simulink model "NoC_4x4x3"  (R2015a)
settings: Solver=ode45  StartTime=0.0  StopTime=10.0  RelTol=1e-3
undefined symbols (not defined in the file or in its folder): des, SELECT
undefined symbols (not defined in the file): MAX, MIN, T
libraries: simulink x48
(part 6 of 12)

== system NoC_4x4x3/LayerDown/PE10 ==
  Cancel Timeout : CancelTimeout
  Constant : Constant  Value=SELECT
  Create Generator Selection Variable : Subsystem  TreatAsAtomicUnit=on
      settings: PropExecContextOutsideSubsystem=on
  DST : EventBasedRandomNumber  Distribution=Arbitrary discrete  minUnid=1  maxUnid=16  numValueUnid=5  valueVecDisc=[1 2 3 4]  probVecDisc=[.25 .25 .25 .25]  Seed=SEED+5
  DST1 : EventBasedRandomNumber  Distribution=Arbitrary discrete  minUnid=1  maxUnid=16  numValueUnid=5  valueVecDisc=[1 2 3 4]  probVecDisc=[.25 .25 .25 .25]  Seed=SEED+50
  DST2 : EventBasedRandomNumber  Distribution=Arbitrary discrete  minUnid=1  maxUnid=16  numValueUnid=5  valueVecDisc=[1 2 3 4]  probVecDisc=[.25 .25 .25 .25]  Seed=SEED+500
  Enabled Gate : EnabledGate
  Entity Departure Event to Function-Call Event : EntityDepartureFunctionCallGenerator
  Entity Sink : EntitySink
  Entity Sink1 : EntitySink
  Entity Sink2 : EntitySink
  Generator 1 : TimeBasedEntityGenerator  Distribution=Exponential  Period=.1  InitialSeed=SEED+10  Maximum=.2  Mean=B  ResponseWhenUnblocked=Delayed restart  EntityType=Standard
  Infinite Server : InfiniteServer  ServiceTime=D  EnableTOPort=on
  Input Switch : InputSwitch  SwitchingCriterion=From signal port p
  Schedule Timeout : ScheduleTimeout  TimeoutInterval=D
  Set Attribute : SetAttribute  AttributeName=DST_X|DST_Y|DST_Z  AttributeFrom=Signal port|Signal port|Signal port  AttributeValue=16|1|1  AttributeTreatAsVector=0|1|1  EvaluatedAttributeValue={ [];[];[]}
      settings: InputPortMap=u0,u1,u2
  Start Timer : StartTimer  TimerTag=Departure
  Time-Based Entity Generator : TimeBasedEntityGenerator  Distribution=Exponential  Period=15  InitialSeed=51335  Maximum=2  Mean=A  PriorityEntityGeneration=350  EntityType=Standard
  Time-Based Entity Generator1 : TimeBasedEntityGenerator  Period=REGULAR
  Time-Based Entity Generator2 : TimeBasedEntityGenerator  Distribution=Uniform  InitialSeed=54552  Minimum=MINU  Maximum=MAXU
  Data_out : PMIOPort  Port=1  Side=Right
  Data_in : PMIOPort  Port=2  Side=Left
  wires:
  Create Generator Selection Variable/1(Out1) -> Enabled Gate/1
  Entity Departure Event to Function-Call Event/1 -> Create Generator Selection Variable/Trigger
  Constant/1 -> Input Switch/1
  DST/1 -> Set Attribute/1
  DST1/1 -> Set Attribute/2
  DST2/1 -> Set Attribute/3
  connections:
  Entity Departure Event to Function-Call Event/RConn1 -- Entity Sink/LConn1
  Time-Based Entity Generator/RConn1 -- Entity Departure Event to Function-Call Event/LConn1
  Generator 1/RConn1 -- Enabled Gate/LConn1
  Time-Based Entity Generator1/RConn1 -- Input Switch/LConn1
  Input Switch/LConn2 -- Time-Based Entity Generator2/RConn1
  Enabled Gate/RConn1 -- Input Switch/LConn3
  Schedule Timeout/LConn1 -- Set Attribute/RConn1
  Cancel Timeout/LConn1 -- Infinite Server/RConn1
  Set Attribute/LConn1 -- Input Switch/RConn1
  Data_out/RConn1 -- Start Timer/RConn1
  Start Timer/LConn1 -- Cancel Timeout/RConn1
  Entity Sink1/LConn1 -- Data_in/RConn1
  Schedule Timeout/RConn1 -- Infinite Server/LConn1
  Infinite Server/RConn2 -- Entity Sink2/LConn1

== system NoC_4x4x3/LayerDown/PE11 ==
  Constant : Constant  Value=SELECT
  Create Generator Selection Variable : Subsystem  TreatAsAtomicUnit=on
      settings: PropExecContextOutsideSubsystem=on
  DST : EventBasedRandomNumber  Distribution=Arbitrary discrete  minUnid=1  maxUnid=16  numValueUnid=5  valueVecDisc=[1 2 3 4]  probVecDisc=[.25 .25 .25 .25]  Seed=SEED+5
  DST1 : EventBasedRandomNumber  Distribution=Arbitrary discrete  minUnid=1  maxUnid=16  numValueUnid=5  valueVecDisc=[1 2 3 4]  probVecDisc=[.25 .25 .25 .25]  Seed=SEED+50
  DST2 : EventBasedRandomNumber  Distribution=Arbitrary discrete  minUnid=1  maxUnid=16  numValueUnid=5  valueVecDisc=[1 2 3 4]  probVecDisc=[.25 .25 .25 .25]  Seed=SEED+500
  Enabled Gate : EnabledGate
  Entity Departure Event to Function-Call Event : EntityDepartureFunctionCallGenerator
  Entity Sink : EntitySink
  Entity Sink1 : EntitySink
  Generator 1 : TimeBasedEntityGenerator  Distribution=Exponential  Period=.1  InitialSeed=SEED+10  Maximum=.2  Mean=B  ResponseWhenUnblocked=Delayed restart  EntityType=Standard
  Infinite Server : InfiniteServer  ServiceTime=0  StatAverageWait=on
      settings: OutputPortMap=o4
  Input Switch : InputSwitch  SwitchingCriterion=From signal port p  StatNumberDeparted=on
  Loss : ToWorkspace  VariableName=Midlle_Loss_Z1  SaveFormat=Timeseries  SampleTime=-1
  N : ToWorkspace  VariableName=Midlle_N_Z1  SaveFormat=Timeseries  SampleTime=-1
  Read Timer : ReadTimer  TimerTag=Departure  StatAverageTimeElapsed=on
      settings: OutputPortMap=o3
  Router : ToWorkspace  VariableName=Midlle_Mean_Z1  SaveFormat=Timeseries  SampleTime=-1
  Set Attribute : SetAttribute  AttributeName=DST_X|DST_Y|DST_Z  AttributeFrom=Signal port|Signal port|Signal port  AttributeValue=16|1|1  AttributeTreatAsVector=0|1|1  StatNumberDeparted=on  EvaluatedAttributeValue={ [];[];[]}
      settings: InputPortMap=u0,u1,u2
  Start Timer : StartTimer  TimerTag=Departure
  Time-Based Entity Generator : TimeBasedEntityGenerator  Distribution=Exponential  Period=15  InitialSeed=57769  Maximum=2  Mean=A  PriorityEntityGeneration=350  EntityType=Standard
  Time-Based Entity Generator1 : TimeBasedEntityGenerator  Period=REGULAR
  Time-Based Entity Generator2 : TimeBasedEntityGenerator  Distribution=Uniform  InitialSeed=60986  Minimum=MINU  Maximum=MAXU
  Data_out : PMIOPort  Port=1  Side=Right
  Data_in : PMIOPort  Port=2  Side=Left
  wires:
  DST2/1 -> Set Attribute/3
  DST1/1 -> Set Attribute/2
  DST/1 -> Set Attribute/1
  Input Switch/1 -> N/1
  Read Timer/1 -> Router/1
  Constant/1 -> Input Switch/1
  Entity Departure Event to Function-Call Event/1 -> Create Generator Selection Variable/Trigger
  Create Generator Selection Variable/1(Out1) -> Enabled Gate/1
  Infinite Server/1 -> Loss/1
  connections:
  Data_in/RConn1 -- Read Timer/LConn1
  Entity Sink1/LConn1 -- Read Timer/RConn1
  Set Attribute/LConn1 -- Input Switch/RConn1
  Enabled Gate/RConn1 -- Input Switch/LConn3
  Input Switch/LConn2 -- Time-Based Entity Generator2/RConn1
  Time-Based Entity Generator1/RConn1 -- Input Switch/LConn1
  Generator 1/RConn1 -- Enabled Gate/LConn1
  Time-Based Entity Generator/RConn1 -- Entity Departure Event to Function-Call Event/LConn1
  Entity Departure Event to Function-Call Event/RConn1 -- Entity Sink/LConn1
  Start Timer/RConn1 -- Infinite Server/LConn1
  Start Timer/LConn1 -- Set Attribute/RConn1
  Infinite Server/RConn1 -- Data_out/RConn1

== system NoC_4x4x3/LayerDown/PE12 ==
  Cancel Timeout : CancelTimeout
  Constant : Constant  Value=SELECT
  Create Generator Selection Variable : Subsystem  TreatAsAtomicUnit=on
      settings: PropExecContextOutsideSubsystem=on
  DST : EventBasedRandomNumber  Distribution=Arbitrary discrete  minUnid=1  maxUnid=16  numValueUnid=5  valueVecDisc=[1 2 3 4]  probVecDisc=[.25 .25 .25 .25]  Seed=SEED+5
  DST1 : EventBasedRandomNumber  Distribution=Arbitrary discrete  minUnid=1  maxUnid=16  numValueUnid=5  valueVecDisc=[1 2 3 4]  probVecDisc=[.25 .25 .25 .25]  Seed=SEED+50
  DST2 : EventBasedRandomNumber  Distribution=Arbitrary discrete  minUnid=1  maxUnid=16  numValueUnid=5  valueVecDisc=[1 2 3 4]  probVecDisc=[.25 .25 .25 .25]  Seed=SEED+500
  Enabled Gate : EnabledGate
  Entity Departure Event to Function-Call Event : EntityDepartureFunctionCallGenerator
  Entity Sink : EntitySink
  Entity Sink1 : EntitySink
  Entity Sink2 : EntitySink
  Generator 1 : TimeBasedEntityGenerator  Distribution=Exponential  Period=.1  InitialSeed=SEED+10  Maximum=.2  Mean=B  ResponseWhenUnblocked=Delayed restart  EntityType=Standard
  Infinite Server : InfiniteServer  ServiceTime=D  EnableTOPort=on
  Input Switch : InputSwitch  SwitchingCriterion=From signal port p
  Schedule Timeout : ScheduleTimeout  TimeoutInterval=D
  Set Attribute : SetAttribute  AttributeName=DST_X|DST_Y|DST_Z  AttributeFrom=Signal port|Signal port|Signal port  AttributeValue=16|1|1  AttributeTreatAsVector=0|1|1  EvaluatedAttributeValue={ [];[];[]}
      settings: InputPortMap=u0,u1,u2
  Start Timer : StartTimer  TimerTag=Departure
  Time-Based Entity Generator : TimeBasedEntityGenerator  Distribution=Exponential  Period=15  InitialSeed=64203  Maximum=2  Mean=A  PriorityEntityGeneration=350  EntityType=Standard
  Time-Based Entity Generator1 : TimeBasedEntityGenerator  Period=REGULAR
  Time-Based Entity Generator2 : TimeBasedEntityGenerator  Distribution=Uniform  InitialSeed=1884  Minimum=MINU  Maximum=MAXU
  Data_out : PMIOPort  Port=1  Side=Right
  Data_in : PMIOPort  Port=2  Side=Left
  wires:
  DST2/1 -> Set Attribute/3
  DST1/1 -> Set Attribute/2
  DST/1 -> Set Attribute/1
  Constant/1 -> Input Switch/1
  Entity Departure Event to Function-Call Event/1 -> Create Generator Selection Variable/Trigger
  Create Generator Selection Variable/1(Out1) -> Enabled Gate/1
  connections:
  Infinite Server/RConn2 -- Entity Sink2/LConn1
  Schedule Timeout/RConn1 -- Infinite Server/LConn1
  Entity Sink1/LConn1 -- Data_in/RConn1
  Start Timer/LConn1 -- Cancel Timeout/RConn1
  Data_out/RConn1 -- Start Timer/RConn1
  Set Attribute/LConn1 -- Input Switch/RConn1
  Cancel Timeout/LConn1 -- Infinite Server/RConn1
  Schedule Timeout/LConn1 -- Set Attribute/RConn1
  Enabled Gate/RConn1 -- Input Switch/LConn3
  Input Switch/LConn2 -- Time-Based Entity Generator2/RConn1
  Time-Based Entity Generator1/RConn1 -- Input Switch/LConn1
  Generator 1/RConn1 -- Enabled Gate/LConn1
  Time-Based Entity Generator/RConn1 -- Entity Departure Event to Function-Call Event/LConn1
  Entity Departure Event to Function-Call Event/RConn1 -- Entity Sink/LConn1

== system NoC_4x4x3/LayerDown/PE13 ==
  Cancel Timeout : CancelTimeout
  Constant : Constant  Value=SELECT
  Create Generator Selection Variable : Subsystem  TreatAsAtomicUnit=on
      settings: PropExecContextOutsideSubsystem=on
  DST : EventBasedRandomNumber  Distribution=Arbitrary discrete  minUnid=1  maxUnid=16  numValueUnid=5  valueVecDisc=[1 2 3 4]  probVecDisc=[.25 .25 .25 .25]  Seed=SEED+5
  DST1 : EventBasedRandomNumber  Distribution=Arbitrary discrete  minUnid=1  maxUnid=16  numValueUnid=5  valueVecDisc=[1 2 3 4]  probVecDisc=[.25 .25 .25 .25]  Seed=SEED+50
  DST2 : EventBasedRandomNumber  Distribution=Arbitrary discrete  minUnid=1  maxUnid=16  numValueUnid=5  valueVecDisc=[1 2 3 4]  probVecDisc=[.25 .25 .25 .25]  Seed=SEED+500
  Enabled Gate : EnabledGate
  Entity Departure Event to Function-Call Event : EntityDepartureFunctionCallGenerator
  Entity Sink : EntitySink
  Entity Sink1 : EntitySink
  Entity Sink2 : EntitySink
  Generator 1 : TimeBasedEntityGenerator  Distribution=Exponential  Period=.1  InitialSeed=SEED+10  Maximum=.2  Mean=B  ResponseWhenUnblocked=Delayed restart  EntityType=Standard
  Infinite Server : InfiniteServer  ServiceTime=D  EnableTOPort=on
  Input Switch : InputSwitch  SwitchingCriterion=From signal port p
  Schedule Timeout : ScheduleTimeout  TimeoutInterval=D
  Set Attribute : SetAttribute  AttributeName=DST_X|DST_Y|DST_Z  AttributeFrom=Signal port|Signal port|Signal port  AttributeValue=16|1|1  AttributeTreatAsVector=0|1|1  EvaluatedAttributeValue={ [];[];[]}
      settings: InputPortMap=u0,u1,u2
  Start Timer : StartTimer  TimerTag=Departure
  Time-Based Entity Generator : TimeBasedEntityGenerator  Distribution=Exponential  Period=15  InitialSeed=5101  Maximum=2  Mean=A  PriorityEntityGeneration=350  EntityType=Standard
  Time-Based Entity Generator1 : TimeBasedEntityGenerator  Period=REGULAR
  Time-Based Entity Generator2 : TimeBasedEntityGenerator  Distribution=Uniform  InitialSeed=8318  Minimum=MINU  Maximum=MAXU
  Data_out : PMIOPort  Port=1  Side=Right
  Data_in : PMIOPort  Port=2  Side=Left
  wires:
  Create Generator Selection Variable/1(Out1) -> Enabled Gate/1
  Entity Departure Event to Function-Call Event/1 -> Create Generator Selection Variable/Trigger
  Constant/1 -> Input Switch/1
  DST/1 -> Set Attribute/1
  DST1/1 -> Set Attribute/2
  DST2/1 -> Set Attribute/3
  connections:
  Entity Departure Event to Function-Call Event/RConn1 -- Entity Sink/LConn1
  Time-Based Entity Generator/RConn1 -- Entity Departure Event to Function-Call Event/LConn1
  Generator 1/RConn1 -- Enabled Gate/LConn1
  Time-Based Entity Generator1/RConn1 -- Input Switch/LConn1
  Input Switch/LConn2 -- Time-Based Entity Generator2/RConn1
  Enabled Gate/RConn1 -- Input Switch/LConn3
  Schedule Timeout/LConn1 -- Set Attribute/RConn1
  Cancel Timeout/LConn1 -- Infinite Server/RConn1
  Set Attribute/LConn1 -- Input Switch/RConn1
  Data_out/RConn1 -- Start Timer/RConn1
  Start Timer/LConn1 -- Cancel Timeout/RConn1
  Entity Sink1/LConn1 -- Data_in/RConn1
  Schedule Timeout/RConn1 -- Infinite Server/LConn1
  Infinite Server/RConn2 -- Entity Sink2/LConn1

== system NoC_4x4x3/LayerDown/PE20 ==
  Cancel Timeout : CancelTimeout
  Constant : Constant  Value=SELECT
  Create Generator Selection Variable : Subsystem  TreatAsAtomicUnit=on
      settings: PropExecContextOutsideSubsystem=on
  DST : EventBasedRandomNumber  Distribution=Arbitrary discrete  minUnid=1  maxUnid=16  numValueUnid=5  valueVecDisc=[1 2 3 4]  probVecDisc=[.25 .25 .25 .25]  Seed=SEED+5
  DST1 : EventBasedRandomNumber  Distribution=Arbitrary discrete  minUnid=1  maxUnid=16  numValueUnid=5  valueVecDisc=[1 2 3 4]  probVecDisc=[.25 .25 .25 .25]  Seed=SEED+50
  DST2 : EventBasedRandomNumber  Distribution=Arbitrary discrete  minUnid=1  maxUnid=16  numValueUnid=5  valueVecDisc=[1 2 3 4]  probVecDisc=[.25 .25 .25 .25]  Seed=SEED+500
  Enabled Gate : EnabledGate
  Entity Departure Event to Function-Call Event : EntityDepartureFunctionCallGenerator
  Entity Sink : EntitySink
  Entity Sink1 : EntitySink
  Entity Sink2 : EntitySink
  Generator 1 : TimeBasedEntityGenerator  Distribution=Exponential  Period=.1  InitialSeed=SEED+10  Maximum=.2  Mean=B  ResponseWhenUnblocked=Delayed restart  EntityType=Standard
  Infinite Server : InfiniteServer  ServiceTime=D  EnableTOPort=on
  Input Switch : InputSwitch  SwitchingCriterion=From signal port p
  Schedule Timeout : ScheduleTimeout  TimeoutInterval=D
  Set Attribute : SetAttribute  AttributeName=DST_X|DST_Y|DST_Z  AttributeFrom=Signal port|Signal port|Signal port  AttributeValue=16|1|1  AttributeTreatAsVector=0|1|1  EvaluatedAttributeValue={ [];[];[]}
      settings: InputPortMap=u0,u1,u2
  Start Timer : StartTimer  TimerTag=Departure
  Time-Based Entity Generator : TimeBasedEntityGenerator  Distribution=Exponential  Period=15  InitialSeed=11535  Maximum=2  Mean=A  PriorityEntityGeneration=350  EntityType=Standard
  Time-Based Entity Generator1 : TimeBasedEntityGenerator  Period=REGULAR
  Time-Based Entity Generator2 : TimeBasedEntityGenerator  Distribution=Uniform  InitialSeed=14752  Minimum=MINU  Maximum=MAXU
  Data_out : PMIOPort  Port=1  Side=Right
  Data_in : PMIOPort  Port=2  Side=Left
  wires:
  DST2/1 -> Set Attribute/3
  DST1/1 -> Set Attribute/2
  DST/1 -> Set Attribute/1
  Constant/1 -> Input Switch/1
  Entity Departure Event to Function-Call Event/1 -> Create Generator Selection Variable/Trigger
  Create Generator Selection Variable/1(Out1) -> Enabled Gate/1
  connections:
  Infinite Server/RConn2 -- Entity Sink2/LConn1
  Schedule Timeout/RConn1 -- Infinite Server/LConn1
  Entity Sink1/LConn1 -- Data_in/RConn1
  Start Timer/LConn1 -- Cancel Timeout/RConn1
  Data_out/RConn1 -- Start Timer/RConn1
  Set Attribute/LConn1 -- Input Switch/RConn1
  Cancel Timeout/LConn1 -- Infinite Server/RConn1
  Schedule Timeout/LConn1 -- Set Attribute/RConn1
  Enabled Gate/RConn1 -- Input Switch/LConn3
  Input Switch/LConn2 -- Time-Based Entity Generator2/RConn1
  Time-Based Entity Generator1/RConn1 -- Input Switch/LConn1
  Generator 1/RConn1 -- Enabled Gate/LConn1
  Time-Based Entity Generator/RConn1 -- Entity Departure Event to Function-Call Event/LConn1
  Entity Departure Event to Function-Call Event/RConn1 -- Entity Sink/LConn1

== system NoC_4x4x3/LayerDown/PE21 ==
  Cancel Timeout : CancelTimeout
  Constant : Constant  Value=SELECT
  Create Generator Selection Variable : Subsystem  TreatAsAtomicUnit=on
      settings: PropExecContextOutsideSubsystem=on
  DST : EventBasedRandomNumber  Distribution=Arbitrary discrete  minUnid=1  maxUnid=16  numValueUnid=5  valueVecDisc=[1 2 3 4]  probVecDisc=[.25 .25 .25 .25]  Seed=SEED+5
  DST1 : EventBasedRandomNumber  Distribution=Arbitrary discrete  minUnid=1  maxUnid=16  numValueUnid=5  valueVecDisc=[1 2 3 4]  probVecDisc=[.25 .25 .25 .25]  Seed=SEED+50
  DST2 : EventBasedRandomNumber  Distribution=Arbitrary discrete  minUnid=1  maxUnid=16  numValueUnid=5  valueVecDisc=[1 2 3 4]  probVecDisc=[.25 .25 .25 .25]  Seed=SEED+500
  Enabled Gate : EnabledGate
  Entity Departure Event to Function-Call Event : EntityDepartureFunctionCallGenerator
  Entity Sink : EntitySink
  Entity Sink1 : EntitySink
  Entity Sink2 : EntitySink
  Generator 1 : TimeBasedEntityGenerator  Distribution=Exponential  Period=.1  InitialSeed=SEED+10  Maximum=.2  Mean=B  ResponseWhenUnblocked=Delayed restart  EntityType=Standard
  Infinite Server : InfiniteServer  ServiceTime=D  EnableTOPort=on
  Input Switch : InputSwitch  SwitchingCriterion=From signal port p
  Schedule Timeout : ScheduleTimeout  TimeoutInterval=D
  Set Attribute : SetAttribute  AttributeName=DST_X|DST_Y|DST_Z  AttributeFrom=Signal port|Signal port|Signal port  AttributeValue=16|1|1  AttributeTreatAsVector=0|1|1  EvaluatedAttributeValue={ [];[];[]}
      settings: InputPortMap=u0,u1,u2
  Start Timer : StartTimer  TimerTag=Departure
  Time-Based Entity Generator : TimeBasedEntityGenerator  Distribution=Exponential  Period=15  InitialSeed=17969  Maximum=2  Mean=A  PriorityEntityGeneration=350  EntityType=Standard
  Time-Based Entity Generator1 : TimeBasedEntityGenerator  Period=REGULAR
  Time-Based Entity Generator2 : TimeBasedEntityGenerator  Distribution=Uniform  InitialSeed=21186  Minimum=MINU  Maximum=MAXU
  Data_out : PMIOPort  Port=1  Side=Right
  Data_in : PMIOPort  Port=2  Side=Left
  wires:
  Create Generator Selection Variable/1(Out1) -> Enabled Gate/1
  Entity Departure Event to Function-Call Event/1 -> Create Generator Selection Variable/Trigger
  Constant/1 -> Input Switch/1
  DST/1 -> Set Attribute/1
  DST1/1 -> Set Attribute/2
  DST2/1 -> Set Attribute/3
  connections:
  Entity Departure Event to Function-Call Event/RConn1 -- Entity Sink/LConn1
  Time-Based Entity Generator/RConn1 -- Entity Departure Event to Function-Call Event/LConn1
  Generator 1/RConn1 -- Enabled Gate/LConn1
  Time-Based Entity Generator1/RConn1 -- Input Switch/LConn1
  Input Switch/LConn2 -- Time-Based Entity Generator2/RConn1
  Enabled Gate/RConn1 -- Input Switch/LConn3
  Schedule Timeout/LConn1 -- Set Attribute/RConn1
  Cancel Timeout/LConn1 -- Infinite Server/RConn1
  Set Attribute/LConn1 -- Input Switch/RConn1
  Data_out/RConn1 -- Start Timer/RConn1
  Start Timer/LConn1 -- Cancel Timeout/RConn1
  Entity Sink1/LConn1 -- Data_in/RConn1
  Schedule Timeout/RConn1 -- Infinite Server/LConn1
  Infinite Server/RConn2 -- Entity Sink2/LConn1

== system NoC_4x4x3/LayerDown/PE22 ==
  Cancel Timeout : CancelTimeout
  Constant : Constant  Value=SELECT
  Create Generator Selection Variable : Subsystem  TreatAsAtomicUnit=on
      settings: PropExecContextOutsideSubsystem=on
  DST : EventBasedRandomNumber  Distribution=Arbitrary discrete  minUnid=1  maxUnid=16  numValueUnid=5  valueVecDisc=[1 2 3 4]  probVecDisc=[.25 .25 .25 .25]  Seed=SEED+5
  DST1 : EventBasedRandomNumber  Distribution=Arbitrary discrete  minUnid=1  maxUnid=16  numValueUnid=5  valueVecDisc=[1 2 3 4]  probVecDisc=[.25 .25 .25 .25]  Seed=SEED+50
  DST2 : EventBasedRandomNumber  Distribution=Arbitrary discrete  minUnid=1  maxUnid=16  numValueUnid=5  valueVecDisc=[1 2 3 4]  probVecDisc=[.25 .25 .25 .25]  Seed=SEED+500
  Enabled Gate : EnabledGate
  Entity Departure Event to Function-Call Event : EntityDepartureFunctionCallGenerator
  Entity Sink : EntitySink
  Entity Sink1 : EntitySink
  Entity Sink2 : EntitySink
  Generator 1 : TimeBasedEntityGenerator  Distribution=Exponential  Period=.1  InitialSeed=SEED+10  Maximum=.2  Mean=B  ResponseWhenUnblocked=Delayed restart  EntityType=Standard
  Infinite Server : InfiniteServer  ServiceTime=D  EnableTOPort=on
  Input Switch : InputSwitch  SwitchingCriterion=From signal port p
  Schedule Timeout : ScheduleTimeout  TimeoutInterval=D
  Set Attribute : SetAttribute  AttributeName=DST_X|DST_Y|DST_Z  AttributeFrom=Signal port|Signal port|Signal port  AttributeValue=16|1|1  AttributeTreatAsVector=0|1|1  EvaluatedAttributeValue={ [];[];[]}
      settings: InputPortMap=u0,u1,u2
  Start Timer : StartTimer  TimerTag=Departure
  Time-Based Entity Generator : TimeBasedEntityGenerator  Distribution=Exponential  Period=15  InitialSeed=24403  Maximum=2  Mean=A  PriorityEntityGeneration=350  EntityType=Standard
  Time-Based Entity Generator1 : TimeBasedEntityGenerator  Period=REGULAR
  Time-Based Entity Generator2 : TimeBasedEntityGenerator  Distribution=Uniform  InitialSeed=27620  Minimum=MINU  Maximum=MAXU
  Data_out : PMIOPort  Port=1  Side=Right
  Data_in : PMIOPort  Port=2  Side=Left
  wires:
  Create Generator Selection Variable/1(Out1) -> Enabled Gate/1
  Entity Departure Event to Function-Call Event/1 -> Create Generator Selection Variable/Trigger
  Constant/1 -> Input Switch/1
  DST/1 -> Set Attribute/1
  DST1/1 -> Set Attribute/2
  DST2/1 -> Set Attribute/3
  connections:
  Entity Departure Event to Function-Call Event/RConn1 -- Entity Sink/LConn1
  Time-Based Entity Generator/RConn1 -- Entity Departure Event to Function-Call Event/LConn1
  Generator 1/RConn1 -- Enabled Gate/LConn1
  Time-Based Entity Generator1/RConn1 -- Input Switch/LConn1
  Input Switch/LConn2 -- Time-Based Entity Generator2/RConn1
  Enabled Gate/RConn1 -- Input Switch/LConn3
  Schedule Timeout/LConn1 -- Set Attribute/RConn1
  Cancel Timeout/LConn1 -- Infinite Server/RConn1
  Set Attribute/LConn1 -- Input Switch/RConn1
  Data_out/RConn1 -- Start Timer/RConn1
  Start Timer/LConn1 -- Cancel Timeout/RConn1
  Entity Sink1/LConn1 -- Data_in/RConn1
  Schedule Timeout/RConn1 -- Infinite Server/LConn1
  Infinite Server/RConn2 -- Entity Sink2/LConn1

== system NoC_4x4x3/LayerDown/PE23 ==
  Cancel Timeout : CancelTimeout
  Constant : Constant  Value=SELECT
  Create Generator Selection Variable : Subsystem  TreatAsAtomicUnit=on
      settings: PropExecContextOutsideSubsystem=on
  DST : EventBasedRandomNumber  Distribution=Arbitrary discrete  minUnid=1  maxUnid=16  numValueUnid=5  valueVecDisc=[1 2 3 4]  probVecDisc=[.25 .25 .25 .25]  Seed=SEED+5
  DST1 : EventBasedRandomNumber  Distribution=Arbitrary discrete  minUnid=1  maxUnid=16  numValueUnid=5  valueVecDisc=[1 2 3 4]  probVecDisc=[.25 .25 .25 .25]  Seed=SEED+50
  DST2 : EventBasedRandomNumber  Distribution=Arbitrary discrete  minUnid=1  maxUnid=16  numValueUnid=5  valueVecDisc=[1 2 3 4]  probVecDisc=[.25 .25 .25 .25]  Seed=SEED+500
  Enabled Gate : EnabledGate
  Entity Departure Event to Function-Call Event : EntityDepartureFunctionCallGenerator
  Entity Sink : EntitySink
  Entity Sink1 : EntitySink
  Entity Sink2 : EntitySink
  Generator 1 : TimeBasedEntityGenerator  Distribution=Exponential  Period=.1  InitialSeed=SEED+10  Maximum=.2  Mean=B  ResponseWhenUnblocked=Delayed restart  EntityType=Standard
  Infinite Server : InfiniteServer  ServiceTime=D  EnableTOPort=on
  Input Switch : InputSwitch  SwitchingCriterion=From signal port p
  Schedule Timeout : ScheduleTimeout  TimeoutInterval=D
  Set Attribute : SetAttribute  AttributeName=DST_X|DST_Y|DST_Z  AttributeFrom=Signal port|Signal port|Signal port  AttributeValue=16|1|1  AttributeTreatAsVector=0|1|1  EvaluatedAttributeValue={ [];[];[]}
      settings: InputPortMap=u0,u1,u2
  Start Timer : StartTimer  TimerTag=Departure
  Time-Based Entity Generator : TimeBasedEntityGenerator  Distribution=Exponential  Period=15  InitialSeed=30837  Maximum=2  Mean=A  PriorityEntityGeneration=350  EntityType=Standard
  Time-Based Entity Generator1 : TimeBasedEntityGenerator  Period=REGULAR
  Time-Based Entity Generator2 : TimeBasedEntityGenerator  Distribution=Uniform  InitialSeed=34054  Minimum=MINU  Maximum=MAXU
  Data_out : PMIOPort  Port=1  Side=Right
  Data_in : PMIOPort  Port=2  Side=Left
  wires:
  DST2/1 -> Set Attribute/3
  DST1/1 -> Set Attribute/2
  DST/1 -> Set Attribute/1
  Constant/1 -> Input Switch/1
  Entity Departure Event to Function-Call Event/1 -> Create Generator Selection Variable/Trigger
  Create Generator Selection Variable/1(Out1) -> Enabled Gate/1
  connections:
  Infinite Server/RConn2 -- Entity Sink2/LConn1
  Schedule Timeout/RConn1 -- Infinite Server/LConn1
  Entity Sink1/LConn1 -- Data_in/RConn1
  Start Timer/LConn1 -- Cancel Timeout/RConn1
  Data_out/RConn1 -- Start Timer/RConn1
  Set Attribute/LConn1 -- Input Switch/RConn1
  Cancel Timeout/LConn1 -- Infinite Server/RConn1
  Schedule Timeout/LConn1 -- Set Attribute/RConn1
  Enabled Gate/RConn1 -- Input Switch/LConn3
  Input Switch/LConn2 -- Time-Based Entity Generator2/RConn1
  Time-Based Entity Generator1/RConn1 -- Input Switch/LConn1
  Generator 1/RConn1 -- Enabled Gate/LConn1
  Time-Based Entity Generator/RConn1 -- Entity Departure Event to Function-Call Event/LConn1
  Entity Departure Event to Function-Call Event/RConn1 -- Entity Sink/LConn1

== system NoC_4x4x3/LayerDown/PE30 ==
  Cancel Timeout : CancelTimeout
  Constant : Constant  Value=SELECT
  Create Generator Selection Variable : Subsystem  TreatAsAtomicUnit=on
      settings: PropExecContextOutsideSubsystem=on
  DST : EventBasedRandomNumber  Distribution=Arbitrary discrete  minUnid=1  maxUnid=16  numValueUnid=5  valueVecDisc=[1 2 3 4]  probVecDisc=[.25 .25 .25 .25]  Seed=SEED+5
  DST1 : EventBasedRandomNumber  Distribution=Arbitrary discrete  minUnid=1  maxUnid=16  numValueUnid=5  valueVecDisc=[1 2 3 4]  probVecDisc=[.25 .25 .25 .25]  Seed=SEED+50
  DST2 : EventBasedRandomNumber  Distribution=Arbitrary discrete  minUnid=1  maxUnid=16  numValueUnid=5  valueVecDisc=[1 2 3 4]  probVecDisc=[.25 .25 .25 .25]  Seed=SEED+500
  Enabled Gate : EnabledGate
  Entity Departure Event to Function-Call Event : EntityDepartureFunctionCallGenerator
  Entity Sink : EntitySink
  Entity Sink1 : EntitySink
  Entity Sink2 : EntitySink
  Generator 1 : TimeBasedEntityGenerator  Distribution=Exponential  Period=.1  InitialSeed=SEED+10  Maximum=.2  Mean=B  ResponseWhenUnblocked=Delayed restart  EntityType=Standard
  Infinite Server : InfiniteServer  ServiceTime=D  EnableTOPort=on
  Input Switch : InputSwitch  SwitchingCriterion=From signal port p
  Schedule Timeout : ScheduleTimeout  TimeoutInterval=D
  Set Attribute : SetAttribute  AttributeName=DST_X|DST_Y|DST_Z  AttributeFrom=Signal port|Signal port|Signal port  AttributeValue=16|1|1  AttributeTreatAsVector=0|1|1  EvaluatedAttributeValue={ [];[];[]}
      settings: InputPortMap=u0,u1,u2
  Start Timer : StartTimer  TimerTag=Departure
  Time-Based Entity Generator : TimeBasedEntityGenerator  Distribution=Exponential  Period=15  InitialSeed=37271  Maximum=2  Mean=A  PriorityEntityGeneration=350  EntityType=Standard
  Time-Based Entity Generator1 : TimeBasedEntityGenerator  Period=REGULAR
  Time-Based Entity Generator2 : TimeBasedEntityGenerator  Distribution=Uniform  InitialSeed=40488  Minimum=MINU  Maximum=MAXU
  Data_out : PMIOPort  Port=1  Side=Right
  Data_in : PMIOPort  Port=2  Side=Left
  wires:
  Create Generator Selection Variable/1(Out1) -> Enabled Gate/1
  Entity Departure Event to Function-Call Event/1 -> Create Generator Selection Variable/Trigger
  Constant/1 -> Input Switch/1
  DST/1 -> Set Attribute/1
  DST1/1 -> Set Attribute/2
  DST2/1 -> Set Attribute/3
  connections:
  Entity Departure Event to Function-Call Event/RConn1 -- Entity Sink/LConn1
  Time-Based Entity Generator/RConn1 -- Entity Departure Event to Function-Call Event/LConn1
  Generator 1/RConn1 -- Enabled Gate/LConn1
  Time-Based Entity Generator1/RConn1 -- Input Switch/LConn1
  Input Switch/LConn2 -- Time-Based Entity Generator2/RConn1
  Enabled Gate/RConn1 -- Input Switch/LConn3
  Schedule Timeout/LConn1 -- Set Attribute/RConn1
  Cancel Timeout/LConn1 -- Infinite Server/RConn1
  Set Attribute/LConn1 -- Input Switch/RConn1
  Data_out/RConn1 -- Start Timer/RConn1
  Start Timer/LConn1 -- Cancel Timeout/RConn1
  Entity Sink1/LConn1 -- Data_in/RConn1
  Schedule Timeout/RConn1 -- Infinite Server/LConn1
  Infinite Server/RConn2 -- Entity Sink2/LConn1

== system NoC_4x4x3/LayerDown/PE31 ==
  Cancel Timeout : CancelTimeout
  Constant : Constant  Value=SELECT
  Create Generator Selection Variable : Subsystem  TreatAsAtomicUnit=on
      settings: PropExecContextOutsideSubsystem=on
  DST : EventBasedRandomNumber  Distribution=Arbitrary discrete  minUnid=1  maxUnid=16  numValueUnid=5  valueVecDisc=[1 2 3 4]  probVecDisc=[.25 .25 .25 .25]  Seed=SEED+5
  DST1 : EventBasedRandomNumber  Distribution=Arbitrary discrete  minUnid=1  maxUnid=16  numValueUnid=5  valueVecDisc=[1 2 3 4]  probVecDisc=[.25 .25 .25 .25]  Seed=SEED+50
  DST2 : EventBasedRandomNumber  Distribution=Arbitrary discrete  minUnid=1  maxUnid=16  numValueUnid=5  valueVecDisc=[1 2 3 4]  probVecDisc=[.25 .25 .25 .25]  Seed=SEED+500
  Enabled Gate : EnabledGate
  Entity Departure Event to Function-Call Event : EntityDepartureFunctionCallGenerator
  Entity Sink : EntitySink
  Entity Sink1 : EntitySink
  Entity Sink2 : EntitySink
  Generator 1 : TimeBasedEntityGenerator  Distribution=Exponential  Period=.1  InitialSeed=SEED+10  Maximum=.2  Mean=B  ResponseWhenUnblocked=Delayed restart  EntityType=Standard
  Infinite Server : InfiniteServer  ServiceTime=D  EnableTOPort=on
  Input Switch : InputSwitch  SwitchingCriterion=From signal port p
  Schedule Timeout : ScheduleTimeout  TimeoutInterval=D
  Set Attribute : SetAttribute  AttributeName=DST_X|DST_Y|DST_Z  AttributeFrom=Signal port|Signal port|Signal port  AttributeValue=16|1|1  AttributeTreatAsVector=0|1|1  EvaluatedAttributeValue={ [];[];[]}
      settings: InputPortMap=u0,u1,u2
  Start Timer : StartTimer  TimerTag=Departure
  Time-Based Entity Generator : TimeBasedEntityGenerator  Distribution=Exponential  Period=15  InitialSeed=43705  Maximum=2  Mean=A  PriorityEntityGeneration=350  EntityType=Standard
  Time-Based Entity Generator1 : TimeBasedEntityGenerator  Period=REGULAR
  Time-Based Entity Generator2 : TimeBasedEntityGenerator  Distribution=Uniform  InitialSeed=46922  Minimum=MINU  Maximum=MAXU
  Data_out : PMIOPort  Port=1  Side=Right
  Data_in : PMIOPort  Port=2  Side=Left
  wires:
  DST2/1 -> Set Attribute/3
  DST1/1 -> Set Attribute/2
  DST/1 -> Set Attribute/1
  Constant/1 -> Input Switch/1
  Entity Departure Event to Function-Call Event/1 -> Create Generator Selection Variable/Trigger
  Create Generator Selection Variable/1(Out1) -> Enabled Gate/1
  connections:
  Infinite Server/RConn2 -- Entity Sink2/LConn1
  Schedule Timeout/RConn1 -- Infinite Server/LConn1
  Entity Sink1/LConn1 -- Data_in/RConn1
  Start Timer/LConn1 -- Cancel Timeout/RConn1
  Data_out/RConn1 -- Start Timer/RConn1
  Set Attribute/LConn1 -- Input Switch/RConn1
  Cancel Timeout/LConn1 -- Infinite Server/RConn1
  Schedule Timeout/LConn1 -- Set Attribute/RConn1
  Enabled Gate/RConn1 -- Input Switch/LConn3
  Input Switch/LConn2 -- Time-Based Entity Generator2/RConn1
  Time-Based Entity Generator1/RConn1 -- Input Switch/LConn1
  Generator 1/RConn1 -- Enabled Gate/LConn1
  Time-Based Entity Generator/RConn1 -- Entity Departure Event to Function-Call Event/LConn1
  Entity Departure Event to Function-Call Event/RConn1 -- Entity Sink/LConn1

== system NoC_4x4x3/LayerDown/PE32 ==
  Cancel Timeout : CancelTimeout
  Constant : Constant  Value=SELECT
  Create Generator Selection Variable : Subsystem  TreatAsAtomicUnit=on
      settings: PropExecContextOutsideSubsystem=on
  DST : EventBasedRandomNumber  Distribution=Arbitrary discrete  minUnid=1  maxUnid=16  numValueUnid=5  valueVecDisc=[1 2 3 4]  probVecDisc=[.25 .25 .25 .25]  Seed=SEED+5
  DST1 : EventBasedRandomNumber  Distribution=Arbitrary discrete  minUnid=1  maxUnid=16  numValueUnid=5  valueVecDisc=[1 2 3 4]  probVecDisc=[.25 .25 .25 .25]  Seed=SEED+50
  DST2 : EventBasedRandomNumber  Distribution=Arbitrary discrete  minUnid=1  maxUnid=16  numValueUnid=5  valueVecDisc=[1 2 3 4]  probVecDisc=[.25 .25 .25 .25]  Seed=SEED+500
  Enabled Gate : EnabledGate
  Entity Departure Event to Function-Call Event : EntityDepartureFunctionCallGenerator
  Entity Sink : EntitySink
  Entity Sink1 : EntitySink
  Entity Sink2 : EntitySink
  Generator 1 : TimeBasedEntityGenerator  Distribution=Exponential  Period=.1  InitialSeed=SEED+10  Maximum=.2  Mean=B  ResponseWhenUnblocked=Delayed restart  EntityType=Standard
  Infinite Server : InfiniteServer  ServiceTime=D  EnableTOPort=on
  Input Switch : InputSwitch  SwitchingCriterion=From signal port p
  Schedule Timeout : ScheduleTimeout  TimeoutInterval=D
  Set Attribute : SetAttribute  AttributeName=DST_X|DST_Y|DST_Z  AttributeFrom=Signal port|Signal port|Signal port  AttributeValue=16|1|1  AttributeTreatAsVector=0|1|1  EvaluatedAttributeValue={ [];[];[]}
      settings: InputPortMap=u0,u1,u2
  Start Timer : StartTimer  TimerTag=Departure
  Time-Based Entity Generator : TimeBasedEntityGenerator  Distribution=Exponential  Period=15  InitialSeed=50139  Maximum=2  Mean=A  PriorityEntityGeneration=350  EntityType=Standard
  Time-Based Entity Generator1 : TimeBasedEntityGenerator  Period=REGULAR
  Time-Based Entity Generator2 : TimeBasedEntityGenerator  Distribution=Uniform  InitialSeed=53356  Minimum=MINU  Maximum=MAXU
  Data_out : PMIOPort  Port=1  Side=Right
  Data_in : PMIOPort  Port=2  Side=Left
  wires:
  DST2/1 -> Set Attribute/3
  DST1/1 -> Set Attribute/2
  DST/1 -> Set Attribute/1
  Constant/1 -> Input Switch/1
  Entity Departure Event to Function-Call Event/1 -> Create Generator Selection Variable/Trigger
  Create Generator Selection Variable/1(Out1) -> Enabled Gate/1
  connections:
  Infinite Server/RConn2 -- Entity Sink2/LConn1
  Schedule Timeout/RConn1 -- Infinite Server/LConn1
  Entity Sink1/LConn1 -- Data_in/RConn1
  Start Timer/LConn1 -- Cancel Timeout/RConn1
  Data_out/RConn1 -- Start Timer/RConn1
  Set Attribute/LConn1 -- Input Switch/RConn1
  Cancel Timeout/LConn1 -- Infinite Server/RConn1
  Schedule Timeout/LConn1 -- Set Attribute/RConn1
  Enabled Gate/RConn1 -- Input Switch/LConn3
  Input Switch/LConn2 -- Time-Based Entity Generator2/RConn1
  Time-Based Entity Generator1/RConn1 -- Input Switch/LConn1
  Generator 1/RConn1 -- Enabled Gate/LConn1
  Time-Based Entity Generator/RConn1 -- Entity Departure Event to Function-Call Event/LConn1
  Entity Departure Event to Function-Call Event/RConn1 -- Entity Sink/LConn1

== system NoC_4x4x3/LayerDown/PE33 ==
  Cancel Timeout : CancelTimeout
  Constant : Constant  Value=SELECT
  Create Generator Selection Variable : Subsystem  TreatAsAtomicUnit=on
      settings: PropExecContextOutsideSubsystem=on
  DST : EventBasedRandomNumber  Distribution=Arbitrary discrete  minUnid=1  maxUnid=16  numValueUnid=5  valueVecDisc=[1 2 3 4]  probVecDisc=[.25 .25 .25 .25]  Seed=SEED+5
  DST1 : EventBasedRandomNumber  Distribution=Arbitrary discrete  minUnid=1  maxUnid=16  numValueUnid=5  valueVecDisc=[1 2 3 4]  probVecDisc=[.25 .25 .25 .25]  Seed=SEED+50
  DST2 : EventBasedRandomNumber  Distribution=Arbitrary discrete  minUnid=1  maxUnid=16  numValueUnid=5  valueVecDisc=[1 2 3 4]  probVecDisc=[.25 .25 .25 .25]  Seed=SEED+500
  Enabled Gate : EnabledGate
  Entity Departure Event to Function-Call Event : EntityDepartureFunctionCallGenerator
  Entity Sink : EntitySink
  Entity Sink1 : EntitySink
  Entity Sink2 : EntitySink
  Generator 1 : TimeBasedEntityGenerator  Distribution=Exponential  Period=.1  InitialSeed=SEED+10  Maximum=.2  Mean=B  ResponseWhenUnblocked=Delayed restart  EntityType=Standard
  Infinite Server : InfiniteServer  ServiceTime=D  EnableTOPort=on
  Input Switch : InputSwitch  SwitchingCriterion=From signal port p
  Schedule Timeout : ScheduleTimeout  TimeoutInterval=D
  Set Attribute : SetAttribute  AttributeName=DST_X|DST_Y|DST_Z  AttributeFrom=Signal port|Signal port|Signal port  AttributeValue=16|1|1  AttributeTreatAsVector=0|1|1  EvaluatedAttributeValue={ [];[];[]}
      settings: InputPortMap=u0,u1,u2
  Start Timer : StartTimer  TimerTag=Departure
  Time-Based Entity Generator : TimeBasedEntityGenerator  Distribution=Exponential  Period=15  InitialSeed=56573  Maximum=2  Mean=A  PriorityEntityGeneration=350  EntityType=Standard
  Time-Based Entity Generator1 : TimeBasedEntityGenerator  Period=REGULAR
  Time-Based Entity Generator2 : TimeBasedEntityGenerator  Distribution=Uniform  InitialSeed=59790  Minimum=MINU  Maximum=MAXU
  Data_out : PMIOPort  Port=1  Side=Right
  Data_in : PMIOPort  Port=2  Side=Left
  wires:
  Create Generator Selection Variable/1(Out1) -> Enabled Gate/1
  Entity Departure Event to Function-Call Event/1 -> Create Generator Selection Variable/Trigger
  Constant/1 -> Input Switch/1
  DST/1 -> Set Attribute/1
  DST1/1 -> Set Attribute/2
  DST2/1 -> Set Attribute/3
  connections:
  Entity Departure Event to Function-Call Event/RConn1 -- Entity Sink/LConn1
  Time-Based Entity Generator/RConn1 -- Entity Departure Event to Function-Call Event/LConn1
  Generator 1/RConn1 -- Enabled Gate/LConn1
  Time-Based Entity Generator1/RConn1 -- Input Switch/LConn1
  Input Switch/LConn2 -- Time-Based Entity Generator2/RConn1
  Enabled Gate/RConn1 -- Input Switch/LConn3
  Schedule Timeout/LConn1 -- Set Attribute/RConn1
  Cancel Timeout/LConn1 -- Infinite Server/RConn1
  Set Attribute/LConn1 -- Input Switch/RConn1
  Data_out/RConn1 -- Start Timer/RConn1
  Start Timer/LConn1 -- Cancel Timeout/RConn1
  Entity Sink1/LConn1 -- Data_in/RConn1
  Schedule Timeout/RConn1 -- Infinite Server/LConn1
  Infinite Server/RConn2 -- Entity Sink2/LConn1

== system NoC_4x4x3/LayerDown/Sitch3DXYZ ==
  FIFO Queue{,1..6} (7 alike) : FIFOQueue
  Output Switch1 : OutputSwitch  NumberOutputPorts=7  SwitchingCriterion=From attribute  AttributeName=RT  InitialConditionsOpt=on  InitialConditions=5
  Path Combiner : PathCombiner  NumberInputPorts=7  InputPortPrecedence=Equiprobable  InitialSeed=4648
  RouteXYZ : Subsystem
  Single Server1 : SingleServer  ServiceTime=D  StatNumberDeparted=on
  Out_N : PMIOPort  Port=1  Side=Right
  In_N : PMIOPort  Port=2  Side=Left
  In_S : PMIOPort  Port=3  Side=Left
  Out_S : PMIOPort  Port=4  Side=Right
  In_W : PMIOPort  Port=5  Side=Left
  Out_W : PMIOPort  Port=6  Side=Right
  In_E : PMIOPort  Port=7  Side=Left
  Out_E : PMIOPort  Port=8  Side=Right
  In_U : PMIOPort  Port=9  Side=Left
  Out_U : PMIOPort  Port=10  Side=Right
  In_D : PMIOPort  Port=11  Side=Left
  In_NI : PMIOPort  Port=12  Side=Left
  Out_D : PMIOPort  Port=13  Side=Right
  Out_NI : PMIOPort  Port=14  Side=Right
  connections:
  Single Server1/LConn1 -- RouteXYZ/RConn1
  Path Combiner/RConn1 -- RouteXYZ/LConn1
  FIFO Queue6/LConn1 -- In_NI/RConn1
  FIFO Queue5/LConn1 -- In_D/RConn1
  Output Switch1/RConn7 -- Out_NI/RConn1
  Output Switch1/RConn6 -- Out_D/RConn1
  Path Combiner/LConn7 -- FIFO Queue6/RConn1
  Path Combiner/LConn6 -- FIFO Queue5/RConn1
  Out_U/RConn1 -- Output Switch1/RConn5
  Out_E/RConn1 -- Output Switch1/RConn4
  Out_W/RConn1 -- Output Switch1/RConn3
  Out_S/RConn1 -- Output Switch1/RConn2
  Out_N/RConn1 -- Output Switch1/RConn1
  Path Combiner/LConn5 -- FIFO Queue4/RConn1
  Path Combiner/LConn4 -- FIFO Queue3/RConn1
  Path Combiner/LConn3 -- FIFO Queue2/RConn1
  Path Combiner/LConn2 -- FIFO Queue1/RConn1
  Path Combiner/LConn1 -- FIFO Queue/RConn1
  Output Switch1/LConn1 -- Single Server1/RConn1
  FIFO Queue4/LConn1 -- In_U/RConn1
  FIFO Queue/LConn1 -- In_N/RConn1
  FIFO Queue3/LConn1 -- In_E/RConn1
  FIFO Queue2/LConn1 -- In_W/RConn1
  FIFO Queue1/LConn1 -- In_S/RConn1

== system NoC_4x4x3/LayerDown/Sitch3DXYZ1 ==
  FIFO Queue{,1..6} (7 alike) : FIFOQueue
  Output Switch1 : OutputSwitch  NumberOutputPorts=7  SwitchingCriterion=From attribute  AttributeName=RT  InitialConditionsOpt=on  InitialConditions=5
  Path Combiner : PathCombiner  NumberInputPorts=7  InputPortPrecedence=Equiprobable  InitialSeed=235
  RouteXYZ : Subsystem
  Single Server1 : SingleServer  ServiceTime=D  StatNumberDeparted=on
  Out_N : PMIOPort  Port=1  Side=Right
  In_N : PMIOPort  Port=2  Side=Left
  In_S : PMIOPort  Port=3  Side=Left
  Out_S : PMIOPort  Port=4  Side=Right
  In_W : PMIOPort  Port=5  Side=Left
  Out_W : PMIOPort  Port=6  Side=Right
  In_E : PMIOPort  Port=7  Side=Left
  Out_E : PMIOPort  Port=8  Side=Right
  In_U : PMIOPort  Port=9  Side=Left
  Out_U : PMIOPort  Port=10  Side=Right
  In_D : PMIOPort  Port=11  Side=Left
  In_NI : PMIOPort  Port=12  Side=Left
  Out_D : PMIOPort  Port=13  Side=Right
  Out_NI : PMIOPort  Port=14  Side=Right
  connections:
  FIFO Queue1/LConn1 -- In_S/RConn1
  FIFO Queue2/LConn1 -- In_W/RConn1
  FIFO Queue3/LConn1 -- In_E/RConn1
  FIFO Queue/LConn1 -- In_N/RConn1
  FIFO Queue4/LConn1 -- In_U/RConn1
  Output Switch1/LConn1 -- Single Server1/RConn1
  Path Combiner/LConn1 -- FIFO Queue/RConn1
  Path Combiner/LConn2 -- FIFO Queue1/RConn1
  Path Combiner/LConn3 -- FIFO Queue2/RConn1
  Path Combiner/LConn4 -- FIFO Queue3/RConn1
  Path Combiner/LConn5 -- FIFO Queue4/RConn1
  Out_N/RConn1 -- Output Switch1/RConn1
  Out_S/RConn1 -- Output Switch1/RConn2
  Out_W/RConn1 -- Output Switch1/RConn3
  Out_E/RConn1 -- Output Switch1/RConn4
  Out_U/RConn1 -- Output Switch1/RConn5
  Path Combiner/LConn6 -- FIFO Queue5/RConn1
  Path Combiner/LConn7 -- FIFO Queue6/RConn1
  Output Switch1/RConn6 -- Out_D/RConn1
  Output Switch1/RConn7 -- Out_NI/RConn1
  FIFO Queue5/LConn1 -- In_D/RConn1
  FIFO Queue6/LConn1 -- In_NI/RConn1
  Path Combiner/RConn1 -- RouteXYZ/LConn1
  Single Server1/LConn1 -- RouteXYZ/RConn1

== system NoC_4x4x3/LayerDown/Sitch3DXYZ10 ==
  FIFO Queue{,1..6} (7 alike) : FIFOQueue
  Output Switch1 : OutputSwitch  NumberOutputPorts=7  SwitchingCriterion=From attribute  AttributeName=RT  InitialConditionsOpt=on  InitialConditions=5
  Path Combiner : PathCombiner  NumberInputPorts=7  InputPortPrecedence=Equiprobable  InitialSeed=56120
  RouteXYZ : Subsystem
  Single Server1 : SingleServer  ServiceTime=D  StatNumberDeparted=on
  Out_N : PMIOPort  Port=1  Side=Right
  In_N : PMIOPort  Port=2  Side=Left
  In_S : PMIOPort  Port=3  Side=Left
  Out_S : PMIOPort  Port=4  Side=Right
  In_W : PMIOPort  Port=5  Side=Left
  Out_W : PMIOPort  Port=6  Side=Right
  In_E : PMIOPort  Port=7  Side=Left
  Out_E : PMIOPort  Port=8  Side=Right
  In_U : PMIOPort  Port=9  Side=Left
  Out_U : PMIOPort  Port=10  Side=Right
  In_D : PMIOPort  Port=11  Side=Left
  In_NI : PMIOPort  Port=12  Side=Left
  Out_D : PMIOPort  Port=13  Side=Right
  Out_NI : PMIOPort  Port=14  Side=Right
  connections:
  Single Server1/LConn1 -- RouteXYZ/RConn1
  Path Combiner/RConn1 -- RouteXYZ/LConn1
  FIFO Queue6/LConn1 -- In_NI/RConn1
  FIFO Queue5/LConn1 -- In_D/RConn1
  Output Switch1/RConn7 -- Out_NI/RConn1
  Output Switch1/RConn6 -- Out_D/RConn1
  Path Combiner/LConn7 -- FIFO Queue6/RConn1
  Path Combiner/LConn6 -- FIFO Queue5/RConn1
  Out_U/RConn1 -- Output Switch1/RConn5
  Out_E/RConn1 -- Output Switch1/RConn4
  Out_W/RConn1 -- Output Switch1/RConn3
  Out_S/RConn1 -- Output Switch1/RConn2
  Out_N/RConn1 -- Output Switch1/RConn1
  Path Combiner/LConn5 -- FIFO Queue4/RConn1
  Path Combiner/LConn4 -- FIFO Queue3/RConn1
  Path Combiner/LConn3 -- FIFO Queue2/RConn1
  Path Combiner/LConn2 -- FIFO Queue1/RConn1
  Path Combiner/LConn1 -- FIFO Queue/RConn1
  Output Switch1/LConn1 -- Single Server1/RConn1
  FIFO Queue4/LConn1 -- In_U/RConn1
  FIFO Queue/LConn1 -- In_N/RConn1
  FIFO Queue3/LConn1 -- In_E/RConn1
  FIFO Queue2/LConn1 -- In_W/RConn1
  FIFO Queue1/LConn1 -- In_S/RConn1

== system NoC_4x4x3/LayerDown/Sitch3DXYZ11 ==
  FIFO Queue{,1..6} (7 alike) : FIFOQueue
  Output Switch1 : OutputSwitch  NumberOutputPorts=7  SwitchingCriterion=From attribute  AttributeName=RT  InitialConditionsOpt=on  InitialConditions=5
  Path Combiner : PathCombiner  NumberInputPorts=7  InputPortPrecedence=Equiprobable  InitialSeed=27167
  RouteXYZ : Subsystem
  Single Server1 : SingleServer  ServiceTime=D  StatNumberDeparted=on
  Out_N : PMIOPort  Port=1  Side=Right
  In_N : PMIOPort  Port=2  Side=Left
  In_S : PMIOPort  Port=3  Side=Left
  Out_S : PMIOPort  Port=4  Side=Right
  In_W : PMIOPort  Port=5  Side=Left
  Out_W : PMIOPort  Port=6  Side=Right
  In_E : PMIOPort  Port=7  Side=Left
  Out_E : PMIOPort  Port=8  Side=Right
  In_U : PMIOPort  Port=9  Side=Left
  Out_U : PMIOPort  Port=10  Side=Right
  In_D : PMIOPort  Port=11  Side=Left
  In_NI : PMIOPort  Port=12  Side=Left
  Out_D : PMIOPort  Port=13  Side=Right
  Out_NI : PMIOPort  Port=14  Side=Right
  connections:
  FIFO Queue1/LConn1 -- In_S/RConn1
  FIFO Queue2/LConn1 -- In_W/RConn1
  FIFO Queue3/LConn1 -- In_E/RConn1
  FIFO Queue/LConn1 -- In_N/RConn1
  FIFO Queue4/LConn1 -- In_U/RConn1
  Output Switch1/LConn1 -- Single Server1/RConn1
  Path Combiner/LConn1 -- FIFO Queue/RConn1
  Path Combiner/LConn2 -- FIFO Queue1/RConn1
  Path Combiner/LConn3 -- FIFO Queue2/RConn1
  Path Combiner/LConn4 -- FIFO Queue3/RConn1
  Path Combiner/LConn5 -- FIFO Queue4/RConn1
  Out_N/RConn1 -- Output Switch1/RConn1
  Out_S/RConn1 -- Output Switch1/RConn2
  Out_W/RConn1 -- Output Switch1/RConn3
  Out_E/RConn1 -- Output Switch1/RConn4
  Out_U/RConn1 -- Output Switch1/RConn5
  Path Combiner/LConn6 -- FIFO Queue5/RConn1
  Path Combiner/LConn7 -- FIFO Queue6/RConn1
  Output Switch1/RConn6 -- Out_D/RConn1
  Output Switch1/RConn7 -- Out_NI/RConn1
  FIFO Queue5/LConn1 -- In_D/RConn1
  FIFO Queue6/LConn1 -- In_NI/RConn1
  Path Combiner/RConn1 -- RouteXYZ/LConn1
  Single Server1/LConn1 -- RouteXYZ/RConn1

== system NoC_4x4x3/LayerDown/Sitch3DXYZ12 ==
  FIFO Queue{,1..6} (7 alike) : FIFOQueue
  Output Switch1 : OutputSwitch  NumberOutputPorts=7  SwitchingCriterion=From attribute  AttributeName=RT  InitialConditionsOpt=on  InitialConditions=5
  Path Combiner : PathCombiner  NumberInputPorts=7  InputPortPrecedence=Equiprobable  InitialSeed=43252
  RouteXYZ : Subsystem
  Single Server1 : SingleServer  ServiceTime=D  StatNumberDeparted=on
  Out_N : PMIOPort  Port=1  Side=Right
  In_N : PMIOPort  Port=2  Side=Left
  In_S : PMIOPort  Port=3  Side=Left
  Out_S : PMIOPort  Port=4  Side=Right
  In_W : PMIOPort  Port=5  Side=Left
  Out_W : PMIOPort  Port=6  Side=Right
  In_E : PMIOPort  Port=7  Side=Left
  Out_E : PMIOPort  Port=8  Side=Right
  In_U : PMIOPort  Port=9  Side=Left
  Out_U : PMIOPort  Port=10  Side=Right
  In_D : PMIOPort  Port=11  Side=Left
  In_NI : PMIOPort  Port=12  Side=Left
  Out_D : PMIOPort  Port=13  Side=Right
  Out_NI : PMIOPort  Port=14  Side=Right
  connections:
  FIFO Queue1/LConn1 -- In_S/RConn1
  FIFO Queue2/LConn1 -- In_W/RConn1
  FIFO Queue3/LConn1 -- In_E/RConn1
  FIFO Queue/LConn1 -- In_N/RConn1
  FIFO Queue4/LConn1 -- In_U/RConn1
  Output Switch1/LConn1 -- Single Server1/RConn1
  Path Combiner/LConn1 -- FIFO Queue/RConn1
  Path Combiner/LConn2 -- FIFO Queue1/RConn1
  Path Combiner/LConn3 -- FIFO Queue2/RConn1
  Path Combiner/LConn4 -- FIFO Queue3/RConn1
  Path Combiner/LConn5 -- FIFO Queue4/RConn1
  Out_N/RConn1 -- Output Switch1/RConn1
  Out_S/RConn1 -- Output Switch1/RConn2
  Out_W/RConn1 -- Output Switch1/RConn3
  Out_E/RConn1 -- Output Switch1/RConn4
  Out_U/RConn1 -- Output Switch1/RConn5
  Path Combiner/LConn6 -- FIFO Queue5/RConn1
  Path Combiner/LConn7 -- FIFO Queue6/RConn1
  Output Switch1/RConn6 -- Out_D/RConn1
  Output Switch1/RConn7 -- Out_NI/RConn1
  FIFO Queue5/LConn1 -- In_D/RConn1
  FIFO Queue6/LConn1 -- In_NI/RConn1
  Path Combiner/RConn1 -- RouteXYZ/LConn1
  Single Server1/LConn1 -- RouteXYZ/RConn1

== system NoC_4x4x3/LayerDown/Sitch3DXYZ13 ==
  FIFO Queue{,1..6} (7 alike) : FIFOQueue
  Output Switch1 : OutputSwitch  NumberOutputPorts=7  SwitchingCriterion=From attribute  AttributeName=RT  InitialConditionsOpt=on  InitialConditions=5
  Path Combiner : PathCombiner  NumberInputPorts=7  InputPortPrecedence=Equiprobable  InitialSeed=33601
  RouteXYZ : Subsystem
  Single Server1 : SingleServer  ServiceTime=D  StatNumberDeparted=on
  Out_N : PMIOPort  Port=1  Side=Right
  In_N : PMIOPort  Port=2  Side=Left
  In_S : PMIOPort  Port=3  Side=Left
  Out_S : PMIOPort  Port=4  Side=Right
  In_W : PMIOPort  Port=5  Side=Left
  Out_W : PMIOPort  Port=6  Side=Right
  In_E : PMIOPort  Port=7  Side=Left
  Out_E : PMIOPort  Port=8  Side=Right
  In_U : PMIOPort  Port=9  Side=Left
  Out_U : PMIOPort  Port=10  Side=Right
  In_D : PMIOPort  Port=11  Side=Left
  In_NI : PMIOPort  Port=12  Side=Left
  Out_D : PMIOPort  Port=13  Side=Right
  Out_NI : PMIOPort  Port=14  Side=Right
  connections:
  Single Server1/LConn1 -- RouteXYZ/RConn1
  Path Combiner/RConn1 -- RouteXYZ/LConn1
  FIFO Queue6/LConn1 -- In_NI/RConn1
  FIFO Queue5/LConn1 -- In_D/RConn1
  Output Switch1/RConn7 -- Out_NI/RConn1
  Output Switch1/RConn6 -- Out_D/RConn1
  Path Combiner/LConn7 -- FIFO Queue6/RConn1
  Path Combiner/LConn6 -- FIFO Queue5/RConn1
  Out_U/RConn1 -- Output Switch1/RConn5
  Out_E/RConn1 -- Output Switch1/RConn4
  Out_W/RConn1 -- Output Switch1/RConn3
  Out_S/RConn1 -- Output Switch1/RConn2
  Out_N/RConn1 -- Output Switch1/RConn1
  Path Combiner/LConn5 -- FIFO Queue4/RConn1
  Path Combiner/LConn4 -- FIFO Queue3/RConn1
  Path Combiner/LConn3 -- FIFO Queue2/RConn1
  Path Combiner/LConn2 -- FIFO Queue1/RConn1
  Path Combiner/LConn1 -- FIFO Queue/RConn1
  Output Switch1/LConn1 -- Single Server1/RConn1
  FIFO Queue4/LConn1 -- In_U/RConn1
  FIFO Queue/LConn1 -- In_N/RConn1
  FIFO Queue3/LConn1 -- In_E/RConn1
  FIFO Queue2/LConn1 -- In_W/RConn1
  FIFO Queue1/LConn1 -- In_S/RConn1
